simulink model "pdmModel"  (R2019b)
settings: Solver=FixedStepDiscrete  StartTime=0.0  StopTime=runTime  RelTol=1e-3  EnableMultiTasking=on
values from neighbouring files (symbols this model uses):
  amp = 0.999969482421875    (= 0.999969482422)    [modelInputData.m]
  cicDecFact = pdmMulti    (= 64)    [modelInputData.m]
  cicFirDecFact = 8    [modelInputData.m]
  cicFirNormGain = 1/(2^(log2(cicFirDecFact)*4))    [modelInputData.m]
  cicNormGain = 1/(2^(log2(cicDecFact)*4))    [modelInputData.m]
  firDecFact = 2    [modelInputData.m]
  freq = 1000    [modelInputData.m]
  fsAnalog = 10*fsPdm    (= 30720000)    [modelInputData.m]
  fsPdm = pdmMulti*fs    (= 3072000)    [modelInputData.m]
undefined symbols (not defined in the file or in its folder): designMultirateFIR, dfilt
libraries: dspmlti4 x5, dsparch4 x2, simulink x1
settings Model: MinMaxOverflowLogging=MinMaxAndOverflow  FPTRunName=NoOverride  Creator=Geas  LastModifiedBy=Geas
settings SolverCC: AutoInsertRateTranBlk=on
settings DataIOCC: ReturnWorkspaceOutputs=off
settings DebuggingCC: SignalRangeChecking=warning  SingleTaskRateTransMsg=error  ParameterDowncastMsg=warning  ParameterOverflowMsg=warning  ArithmeticOperatorsInVariantConditions=warning
settings HardwareCC: ProdBitPerLong=64  ProdHWDeviceType=Intel->x86-64 (Mac OS X)  TargetBitPerLong=64  TargetBitPerPointer=64  TargetBitPerSizeT=64  TargetBitPerPtrDiffT=64  TargetLargestAtomicFloat=Float  TargetIntDivRoundTo=Zero  TargetEndianess=LittleEndian  TargetWordSize=64  TargetPreprocMaxBitsSint=128  TargetPreprocMaxBitsUint=128  TargetHWDeviceType=Intel->x86-64 (Mac OS X)
settings SFSimCC: SimUseLocalCustomCode=off  CustomCodeUndefinedFunction=UseInterfaceOnly
settings RTWCC: RTWUseLocalCustomCode=off
settings CodeAppCC: StateflowObjectComments=on

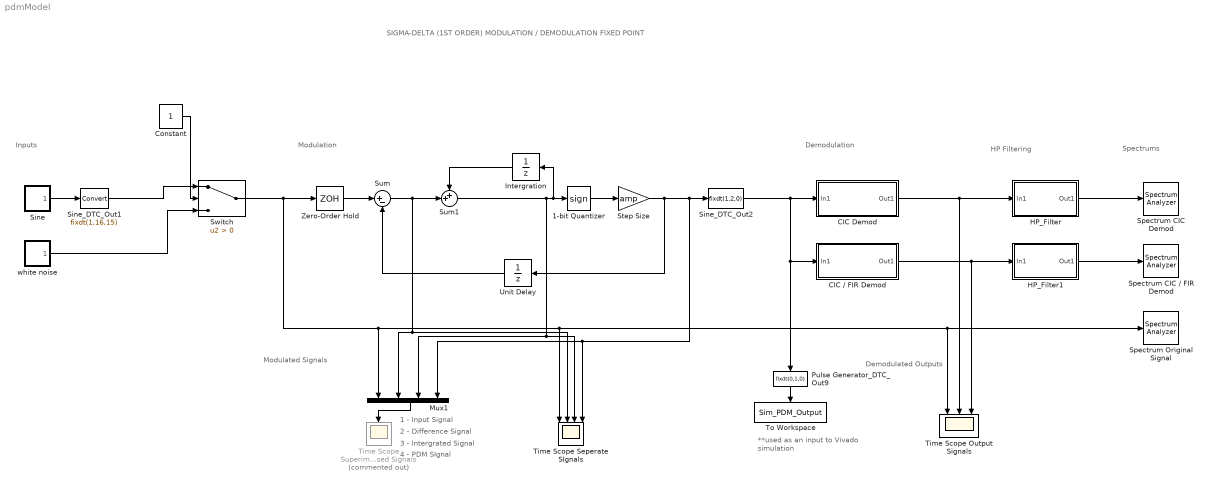
== system pdmModel ==
  note: **used as an input to
      |    Vivado simulation
  note: Inputs
  note: Demodulation
  note: Modulation
  note: Spectrums
  note: Demodulated
      | Outputs
  note: Modulated Signals
  note: 1 - Input Signal
  note: SIGMA-DELTA (1ST ORDER)
      | MODULATION / DEMODULATION
      | FIXED POINT
  note: 2 - Difference Signal
  note: 3 - Intergrated Signal
  note: 4 - PDM SIgnal
  note: HP Filtering
  1-bit Quantizer : Signum
  CIC / FIR Demod : Subsystem
  CIC Demod : Subsystem
  Constant : Constant  OutDataTypeStr=fixdt(0,16,15)
  HP_Filter : Subsystem
  HP_Filter1 : Subsystem
  Intergration : UnitDelay  SampleTime=-1  HasFrameUpgradeWarning=on
  Mux1 : Mux
  Pulse Generator_DTC_Out9 : DataTypeConversion  OutDataTypeStr=fixdt(0,1,0)  RndMeth=Round  SaturateOnIntegerOverflow=on
  Sine : Subsystem  Tag=DecoupledSystem
  Sine_DTC_Out1 : DataTypeConversion  OutDataTypeStr=fixdt(1,16,15)
  Sine_DTC_Out2 : DataTypeConversion  OutDataTypeStr=fixdt(1,2,0)  RndMeth=Round
  Spectrum CIC / FIR Demod : SpectrumAnalyzer
  Spectrum CIC Demod : SpectrumAnalyzer
  Spectrum Original Signal : SpectrumAnalyzer
  Step Size : Gain  Gain=amp  OutDataTypeStr=fixdt(1,16,14)  RndMeth=Round
  Sum : Sum  Inputs=|+-  OutDataTypeStr=fixdt(1,16,14)  RndMeth=Round
  Sum1 : Sum  Inputs=++|  OutDataTypeStr=fixdt(1,16,14)  RndMeth=Round
  Switch : Switch  Criteria=u2 > Threshold  OutDataTypeStr=fixdt(1,16,14)
  Time Scope Output Signals : Scope  NumInputPorts=3
  Time Scope Seperate SIgnals : Scope  NumInputPorts=4
  Time Scope Superimposed Signals : Scope  Commented=on
  To Workspace : ToWorkspace  VariableName=Sim_PDM_Output  SampleTime=1/fsPdm
      settings: Save2DSignal=2-D array (concatenate along first dimension)
  Unit Delay : UnitDelay  SampleTime=-1  HasFrameUpgradeWarning=on
  Zero-Order Hold : ZeroOrderHold  SampleTime=1/fsPdm
  white noise : Subsystem  Tag=DecoupledSystem
  wires:
  Sine/1(Out1) -> Sine_DTC_Out1/1
  Intergration/1 -> Sum1/1
  Sum1/1 -> 1-bit Quantizer/1, Intergration/1, Mux1/3, Time Scope Seperate SIgnals/3
  1-bit Quantizer/1 -> Step Size/1
  Sum/1 -> Sum1/2, Time Scope Seperate SIgnals/2, Mux1/2
  Unit Delay/1 -> Sum/2
  Zero-Order Hold/1 -> Sum/1
  Mux1/1 -> Time Scope Superimposed Signals/1
  CIC Demod/1(Out1) -> HP_Filter/1(In1), Time Scope Output Signals/2
  Sine_DTC_Out2/1 -> CIC Demod/1(In1), CIC / FIR Demod/1(In1), Pulse Generator_DTC_Out9/1
  Switch/1 -> Time Scope Seperate SIgnals/1, Spectrum Original Signal/1, Time Scope Output Signals/1, Mux1/1, Zero-Order Hold/1
  Step Size/1 -> Unit Delay/1, Sine_DTC_Out2/1, Time Scope Seperate SIgnals/4, Mux1/4
  Pulse Generator_DTC_Out9/1 -> To Workspace/1
  CIC / FIR Demod/1(Out1) -> HP_Filter1/1(In1), Time Scope Output Signals/3
  HP_Filter/1(Out1) -> Spectrum CIC Demod/1
  white noise/1(Out1) -> Switch/3
  Sine_DTC_Out1/1 -> Switch/1
  Constant/1 -> Switch/2
  HP_Filter1/1(Out1) -> Spectrum CIC / FIR Demod/1

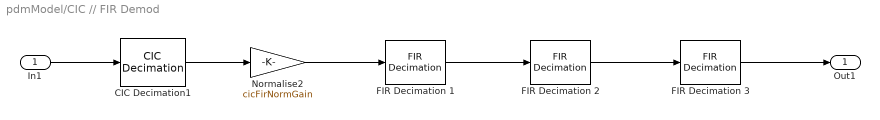
== system pdmModel/CIC // FIR Demod ==
  In1 : Inport  OutDataTypeStr=fixdt(1,2,0)
  CIC Decimation1 : dspmlti4/CIC Decimation  filtFrom=Dialog parameters  filtobj=CICDECIM  ftype=Decimator  R=cicFirDecFact  M=1  N=4  filterInternals=Full precision  BPS=[16 16 16 16]  FLPS=0  outputWordLength=32  outputFracLength=0  launchFVT=off  framing=Maintain input frame rate  RateOptions=Allow multirate processing
      settings: SourceProductName=DSP System Toolbox  SourceProductBaseCode=DS
  FIR Decimation 1 : dspmlti4/FIR Decimation  FilterSource=Auto  h=designMultirateFIR(1,2)  D=firDecFact  filtStruct=Direct form  FilterObject=FDECIM  framing=Enforce single-rate processing  inputOffset=0  outputBufInitCond=0  roundingMode=Floor  overflowMode=off  firstCoeffDataTypeStr=Inherit: Same word length as input  firstCoeffMin=[]  firstCoeffMax=[]  firstCoeffLastDataTypeStr=Inherit: Same word length as input  outputMode=Binary point scaling  outputWordLength=16  outputFracLength=14  outputDataTypeStr=fixdt(1,16,14)  outputMin=[]  outputMax=[]  outputLastDataTypeStr=fixdt(1,16,14)
  FIR Decimation 2 : dspmlti4/FIR Decimation  Tag=FIR 2  FilterSource=Auto  h=designMultirateFIR(1,2)  D=firDecFact  filtStruct=Direct form  FilterObject=FDECIM  framing=Enforce single-rate processing  inputOffset=0  outputBufInitCond=0  roundingMode=Floor  overflowMode=off  firstCoeffDataTypeStr=Inherit: Same word length as input  firstCoeffMin=[]  firstCoeffMax=[]  firstCoeffLastDataTypeStr=Inherit: Same word length as input  outputMode=Binary point scaling  outputWordLength=16  outputFracLength=14  outputDataTypeStr=fixdt(1,16,14)  outputMin=[]  outputMax=[]  outputLastDataTypeStr=fixdt(1,16,14)
  FIR Decimation 3 : dspmlti4/FIR Decimation  FilterSource=Auto  h=designMultirateFIR(1,2)  D=firDecFact  filtStruct=Direct form  FilterObject=FDECIM  framing=Enforce single-rate processing  inputOffset=0  outputBufInitCond=0  roundingMode=Floor  overflowMode=off  firstCoeffDataTypeStr=Inherit: Same word length as input  firstCoeffMin=[]  firstCoeffMax=[]  firstCoeffLastDataTypeStr=Inherit: Same word length as input  outputMode=Binary point scaling  outputWordLength=16  outputFracLength=14  outputDataTypeStr=fixdt(1,16,14)  outputMin=[]  outputMax=[]  outputLastDataTypeStr=fixdt(1,16,14)
  Normalise2 : Gain  Gain=cicFirNormGain  OutDataTypeStr=fixdt(1,16,14)
  Out1 : Outport
  wires:
  In1/1 -> CIC Decimation1/1
  CIC Decimation1/1 -> Normalise2/1
  Normalise2/1 -> FIR Decimation 1/1
  FIR Decimation 1/1 -> FIR Decimation 2/1
  FIR Decimation 2/1 -> FIR Decimation 3/1
  FIR Decimation 3/1 -> Out1/1

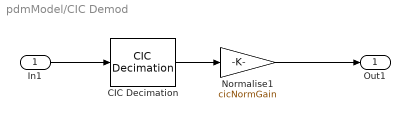
== system pdmModel/CIC Demod ==
  In1 : Inport  OutDataTypeStr=fixdt(1,2,0)
  CIC Decimation : dspmlti4/CIC Decimation  filtFrom=Dialog parameters  filtobj=CICDECIM  ftype=Decimator  R=cicDecFact  M=1  N=4  filterInternals=Full precision  BPS=[16 16 16 16]  FLPS=0  outputWordLength=32  outputFracLength=0  launchFVT=off  framing=Maintain input frame rate  RateOptions=Allow multirate processing
      settings: SourceProductName=DSP System Toolbox  SourceProductBaseCode=DS
  Normalise1 : Gain  Gain=cicNormGain  OutDataTypeStr=fixdt(1,16,14)
  Out1 : Outport
  wires:
  In1/1 -> CIC Decimation/1
  Normalise1/1 -> Out1/1
  CIC Decimation/1 -> Normalise1/1

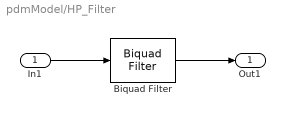
== system pdmModel/HP_Filter ==
  In1 : Inport  OutDataTypeStr=fixdt(1,16,14)
  Biquad Filter : dsparch4/Biquad Filter  FilterSource=Dialog parameters  CoeffSource=Specify via dialog  FilterObject=dfilt.df2tsos([1 0.3 0.4],[1 0.1 0.2])  IIRFiltStruct=Direct form II  BiQuadCoeffs=sosVec  ScaleValues=1  IC=0  ICnum=0  ICden=0  a0Flag=Warning  optimizeScaleValues=on  ScaleValueMode=Specify via input port (g)  roundingMode=Floor  overflowMode=off  stageInputMode=Binary point scaling  stageInputWordLength=32  stageInputFracLength=30  firstCoeffMode=Binary point scaling  firstCoeffWordLength=32  firstCoeffFracLength=30  scaleValueFracLength=1  prodOutputMode=Binary point scaling  prodOutputWordLength=64  prodOutputFracLength=48  denProdOutputFracLength=48  accumMode=Binary point scaling  accumWordLength=64  accumFracLength=48  denAccumFracLength=48  memoryMode=Binary point scaling  memoryWordLength=64  memoryFracLength=48  secondMemoryFracLength=15  outputMode=Binary point scaling  outputWordLength=16  outputFracLength=14
      settings: SourceProductName=DSP System Toolbox
  Out1 : Outport
  wires:
  In1/1 -> Biquad Filter/1
  Biquad Filter/1 -> Out1/1

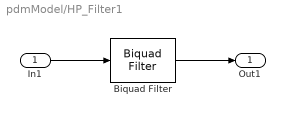
== system pdmModel/HP_Filter1 ==
  In1 : Inport  OutDataTypeStr=fixdt(1,16,14)
  Biquad Filter : dsparch4/Biquad Filter  FilterSource=Dialog parameters  CoeffSource=Specify via dialog  FilterObject=dfilt.df2tsos([1 0.3 0.4],[1 0.1 0.2])  IIRFiltStruct=Direct form II  BiQuadCoeffs=sosVec  ScaleValues=1  IC=0  ICnum=0  ICden=0  a0Flag=Warning  optimizeScaleValues=on  ScaleValueMode=Specify via input port (g)  roundingMode=Floor  overflowMode=off  stageInputMode=Binary point scaling  stageInputWordLength=32  stageInputFracLength=30  firstCoeffMode=Binary point scaling  firstCoeffWordLength=32  firstCoeffFracLength=30  scaleValueFracLength=1  prodOutputMode=Binary point scaling  prodOutputWordLength=64  prodOutputFracLength=48  denProdOutputFracLength=48  accumMode=Binary point scaling  accumWordLength=64  accumFracLength=48  denAccumFracLength=48  memoryMode=Binary point scaling  memoryWordLength=64  memoryFracLength=48  secondMemoryFracLength=15  outputMode=Binary point scaling  outputWordLength=16  outputFracLength=14
      settings: SourceProductName=DSP System Toolbox
  Out1 : Outport
  wires:
  In1/1 -> Biquad Filter/1
  Biquad Filter/1 -> Out1/1

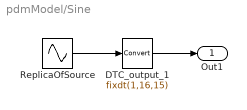
== system pdmModel/Sine ==
  DTC_output_1 : DataTypeConversion  OutDataTypeStr=fixdt(1,16,15)
  ReplicaOfSource : Sin  Amplitude=amp  Frequency=2*pi*freq  SampleTime=1/(fsAnalog)
  Out1 : Outport  LockScale=on
  wires:
  ReplicaOfSource/1 -> DTC_output_1/1
  DTC_output_1/1 -> Out1/1

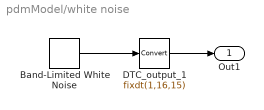
== system pdmModel/white noise ==
  Band-Limited White Noise : simulink/Sources/Band-Limited White Noise  Cov=[2]  Ts=1/(fsAnalog)  seed=[23341]
  DTC_output_1 : DataTypeConversion  OutDataTypeStr=fixdt(1,16,15)
  Out1 : Outport  LockScale=on
  wires:
  DTC_output_1/1 -> Out1/1
  Band-Limited White Noise/1 -> DTC_output_1/1
